simulink model "REALTIME_PART2_nominal"  (R2020b)
settings: Solver=ode3  StartTime=0.0  StopTime=5  FixedStep=0.001  RelTol=1e-3
undefined symbols (not defined in the file or in its folder): degs2rpm, denH1, N_u, N_x, National_Instruments, numH1, PCI, rpm2rads, sens, step_size
libraries: sldrtlib x2
settings Model: ExtModeTrigDuration=6000  Creator=utente  LastModifiedBy=ambrosingi
settings DataIOCC: ReturnWorkspaceOutputs=off
settings RTWCC: Description=Simulink Desktop Real-Time  SystemTargetFile=sldrt.tlc  TemplateMakefile=sldrt.tmf  RTWCompilerOptimization=on
settings CodeAppCC: MaxIdLength=95
settings SimulinkDesktopRealTimeCC: TargetPreCompLibLocation=C:\Program Files\MATLAB\R2020b\toolbox\sldrt\lib\win64

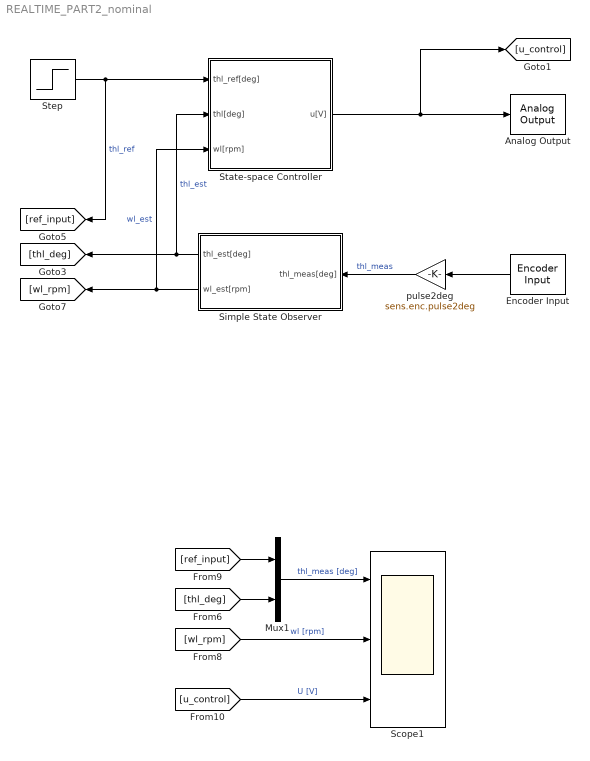
== system REALTIME_PART2_nominal ==
  Analog Output : sldrtlib/Analog Output  SampleTime=0.001  MaxMissedTicks=10  ShowMissedTicks=off  YieldWhenWaiting=off  DrvName=National_Instruments/PCI-6221  DrvAddress=4294967295  DrvOptions=[0 0 0 2 0]  Channels=1  RangeMode=1  VoltRange=1  InitialValue=0  FinalValue=0
      settings: AttributesFormatString=National Instruments\nPCI-6221 [auto]
  Encoder Input : sldrtlib/Encoder Input  SampleTime=0.001  MaxMissedTicks=10  ShowMissedTicks=off  YieldWhenWaiting=off  DrvName=National_Instruments/PCI-6221  DrvAddress=4294967295  DrvOptions=[0 0 0 2 0]  Channels=1  QuadMode=3  IndexPulse=1  InputFilter=Inf  DataType=1
      settings: AttributesFormatString=National Instruments\nPCI-6221 [auto]
  Mux1 : Mux  Inputs=2
  Scope1 : Scope  NumInputPorts=3
  Simple State Observer : Subsystem
  State-space Controller : Subsystem
  Step : Step  After=step_size  SampleTime=0
  pulse2deg : Gain  Gain=sens.enc.pulse2deg
  wires:
  Step/1 -> State-space Controller/1(thl_ref[deg]), [ref_input]  "thl_ref"
  pulse2deg/1 -> Simple State Observer/1(thl_meas[deg])  "thl_meas"
  Simple State Observer/1(thl_est[deg]) -> State-space Controller/2(thl[deg]), [thl_deg]  "thl_est"
  Simple State Observer/2(wl_est[rpm]) -> State-space Controller/3(wl[rpm]), [wl_rpm]  "wl_est"
  State-space Controller/1(u[V]) -> Analog Output/1, [u_control]
  [ref_input] -> Mux1/1
  [u_control] -> Scope1/3  "U [V]"
  Mux1/1 -> Scope1/1  "thl_meas [deg]"
  [thl_deg] -> Mux1/2
  [wl_rpm] -> Scope1/2  "wl [rpm]"
  Encoder Input/1 -> pulse2deg/1

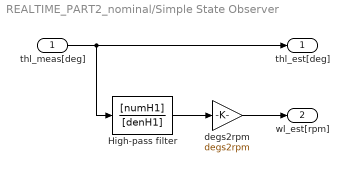
== system REALTIME_PART2_nominal/Simple State Observer ==
  thl_meas[deg] : Inport
  High-pass filter : TransferFcn  Numerator=[numH1]  Denominator=[denH1]
  degs2rpm : Gain  Gain=degs2rpm
  thl_est[deg] : Outport
  wl_est[rpm] : Outport  Port=2
  wires:
  thl_meas[deg]/1 -> thl_est[deg]/1, High-pass filter/1
  High-pass filter/1 -> degs2rpm/1
  degs2rpm/1 -> wl_est[rpm]/1

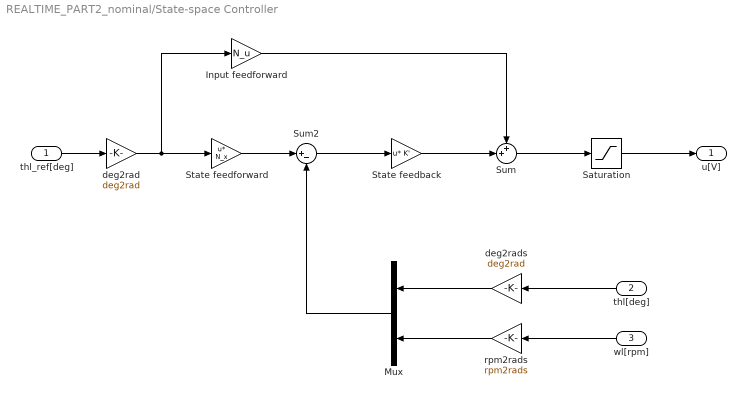
== system REALTIME_PART2_nominal/State-space Controller ==
  thl_ref[deg] : Inport
  thl[deg] : Inport  Port=2
  wl[rpm] : Inport  Port=3
  Input feedforward : Gain  Gain=N_u
  Mux : Mux  Inputs=2
  Saturation : Saturate  UpperLimit=10  LowerLimit=-10
  State feedback : Gain  Gain=K'  Multiplication=Matrix(u*K)
  "State feedforward\t" : Gain  Gain=N_x  Multiplication=Matrix(u*K)
  Sum : Sum  Inputs=++|
  Sum2 : Sum  Inputs=|+-
  deg2rad : Gain  Gain=deg2rad
  deg2rads : Gain  Gain=deg2rad
  rpm2rads : Gain  Gain=rpm2rads
  u[V] : Outport
  wires:
  thl_ref[deg]/1 -> deg2rad/1
  deg2rad/1 -> Input feedforward/1, "State feedforward\t"/1
  State feedback/1 -> Sum/2
  "State feedforward\t"/1 -> Sum2/1
  Sum2/1 -> State feedback/1
  Input feedforward/1 -> Sum/1
  Sum/1 -> Saturation/1
  Saturation/1 -> u[V]/1
  deg2rads/1 -> Mux/1
  rpm2rads/1 -> Mux/2
  thl[deg]/1 -> deg2rads/1
  wl[rpm]/1 -> rpm2rads/1
  Mux/1 -> Sum2/2
